simulink model "Brazoproject"  (R2013a)
settings: Solver=ode45  StartTime=0.0  StopTime=10.0  RelTol=1e-3
values from neighbouring files (symbols this model uses):
  m = [(m1*lc1^2)+m2*(l1^2+lc2^2+2*l1*lc2*cos(q2))+I1+I2 (m2*(lc2^2+l1*lc2*m2*cos(q2)+I2)) ... (first row only)    [brazomire.m]    (also in examvib3.m = 0.2533; fft estatica.m = [0:0.02:100]; fftestatica.m = [0:0.02:100])
undefined symbols (not defined in the file or in its folder): aumento, bacedymami, bacedymamixel, brazo1fribracarbono, brazo2frubra, Ensamblaje1, motordymamixel, par, Pieza1bASE, RootGround, RootPart, soporte, soporteM
libraries: mblibv1 x48
settings Model: Creator=Daniel  LastModifiedBy=Daniel
settings SimMechanicsCC: VisOnUpdateDiagram=on  VisDuringSimulation=on

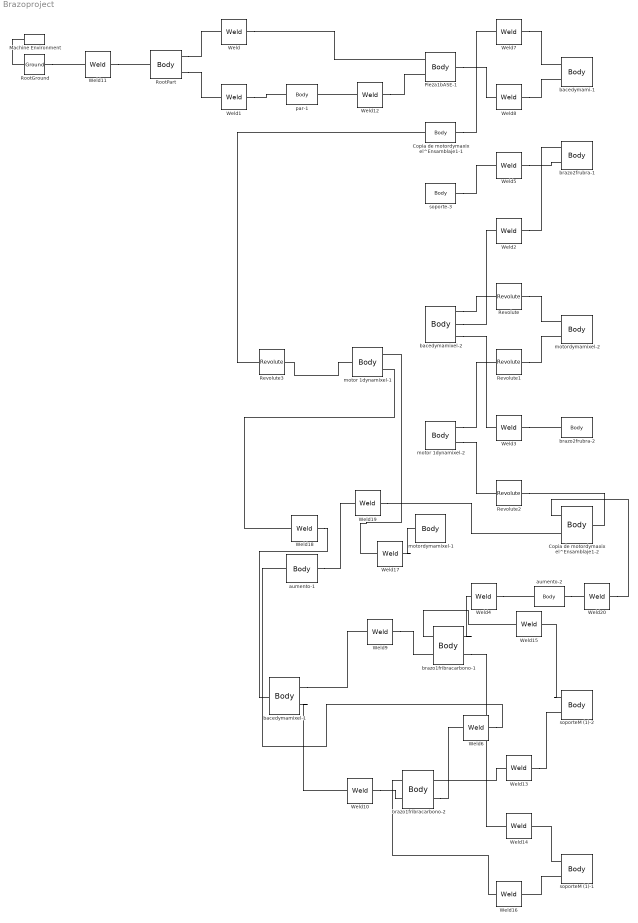
== system Brazoproject ==
  Copia de motordymaxixel^Ensamblaje1-1 : mblibv1/Bodies/Body  LConnTagsString=CS2  RConnTagsString=CS3  UpdateFromCAD=on  PMImportedID=Copia de motordymaxixel^Ensamblaje1-1  DialogClass=MechanicalBodyBlock  Mass=0.038592  MassUnits=kg  InertiaUnits=kg*m^2  Inertia=[1.11428e-05,-9.15437e-14,2.18753e-13;-9.15437e-14,6.03089e-06,1.38272e-07;2.18753e-13,1.38272e-07,9.55884e-06]  Shape=Cylinder  ShapeDims=[1 1]  ShapeUnits=m  ShapeUse=false  Density=1  DensityUnits=kg/m^3  DensityUse=false  GraphicsMode=GFXFILE  GraphicsFileName=Ensamblaje1 - Copia de motordymaxixel^Ensamblaje1-1.STL  BodyColorSelMode=COLORPALETTE  BodyColor=[1;0;0]  AttachedToCS=CS1  CG=Right$CG$[0.0211399 0.214749 0.233224]$WORLD$WORLD$m$[0 0 1;1 0 0;0 1 0]$3x3 Transform$rad$WORLD$false$Copia de motordymaxixel^Ensamblaje1-1::CG(AUTOGEN)  WorkingFrames=Right$CS1$[0.00471859 0.198749 0.20797]$WORLD$WORLD$m$[0 0 1;1 0 0;0 1 0]$3x3 Transform$rad$WORLD$false$Copia de motordymaxixel^Ensamblaje1-1::CS1(AUTOGEN)#Left$CS2$[0.0367186 0.214749 0.24647]$WORLD$WORLD$m$[1 0 0;0 1 0;0 0 1]$3x3 Transform$rad$WORLD$true$Copia de motordymaxixel^Ensamblaje1-1:-:motor 1dynamixel-1::Copia de motordymaxixel^Ensamblaje1-1(AUTOGEN)#Right$CS3$[0.00471859 0.222749 0.21047]$WORLD$WORLD$m$[1 0 0;0 1 0;0 0 1]$3x3 Transform$rad$WORLD$true$Copia de motordymaxixel^Ensamblaje1-1:-:bacedymami-1::Copia de motordymaxixel^Ensamblaje1-1(AUTOGEN)  CGPos=[0.0211399 0.214749 0.233224]  CGRot=[0 0 1;1 0 0;0 1 0]  CS0Pos=[]  CS0Rot=[]  CS1Pos=[0.00471859 0.198749 0.20797]  CS1Rot=[0 0 1;1 0 0;0 1 0]  CS2Pos=[0.0367186 0.214749 0.24647]  CS2Rot=[1 0 0;0 1 0;0 0 1]  CS3Pos=[0.00471859 0.222749 0.21047]  CS3Rot=[1 0 0;0 1 0;0 0 1]  CS4Pos=[]  CS4Rot=[]  CS5Pos=[]  CS5Rot=[]  CS6Pos=[]  CS6Rot=[]  CS7Pos=[]  CS7Rot=[]  CS8Pos=[]  CS8Rot=[]  CS9Pos=[]  CS9Rot=[]  CS10Pos=[]  CS10Rot=[]  CS11Pos=[]  CS11Rot=[]  CS12Pos=[]  CS12Rot=[]  CS13Pos=[]  CS13Rot=[]  CS14Pos=[]  CS14Rot=[]  CS15Pos=[]  CS15Rot=[]  CS16Pos=[]  CS16Rot=[]  CS17Pos=[]  CS17Rot=[]  CS18Pos=[]  CS18Rot=[]  CS19Pos=[]  CS19Rot=[]  CS20Pos=[]  CS20Rot=[]
  Copia de motordymaxixel^Ensamblaje1-2 : mblibv1/Bodies/Body  LConnTagsString=CS1|CS3  RConnTagsString=CS2  UpdateFromCAD=on  PMImportedID=Copia de motordymaxixel^Ensamblaje1-2  DialogClass=MechanicalBodyBlock  Mass=0.038592  MassUnits=kg  InertiaUnits=kg*m^2  Inertia=[1.11428e-05,-9.15437e-14,2.18753e-13;-9.15437e-14,6.03089e-06,1.38272e-07;2.18753e-13,1.38272e-07,9.55884e-06]  Shape=Cylinder  ShapeDims=[1 1]  ShapeUnits=m  ShapeUse=false  Density=1  DensityUnits=kg/m^3  DensityUse=false  GraphicsMode=GFXFILE  GraphicsFileName=Ensamblaje1 - Copia de motordymaxixel^Ensamblaje1-2.STL  BodyColorSelMode=COLORPALETTE  BodyColor=[1 0 0]  AttachedToCS=CS1  CG=Left$CG$[0.0201399 0.341824 0.297002]$WORLD$WORLD$m$[0 0 1;0.36951 0.929227 0;-0.929227 0.36951 0]$3x3 Transform$rad$WORLD$false$Copia de motordymaxixel^Ensamblaje1-2::CG(AUTOGEN)  WorkingFrames=Left$CS1$[0.00371859 0.312445 0.302538]$WORLD$WORLD$m$[0 0 1;0.36951 0.929227 0;-0.929227 0.36951 0]$3x3 Transform$rad$WORLD$true$Copia de motordymaxixel^Ensamblaje1-2::CS1(AUTOGEN)#Right$CS2$[0.0357186 0.354133 0.301897]$WORLD$WORLD$m$[1 0 0;0 1 0;0 0 1]$3x3 Transform$rad$WORLD$true$Copia de motordymaxixel^Ensamblaje1-2:-:motor 1dynamixel-2::Copia de motordymaxixel^Ensamblaje1-2(AUTOGEN)#Left$CS3$[0.00371859 0.198979 0.253651]$WORLD$WORLD$m$[1 0 0;0 1 0;0 0 1]$3x3 Transform$rad$WORLD$true$Copia de motordymaxixel^Ensamblaje1-2:-:aumento-1::Copia de motordymaxixel^Ensamblaje1-2(AUTOGEN)#Left$CS4$[0.00371859 0.317724 0.296028]$WORLD$WORLD$m$[1 0 0;0 1 0;0 0 1]$3x3 Transform$rad$WORLD$false$Copia de motordymaxixel^Ensamblaje1-2:-:brazo1fribracarbono-2::Copia de motordymaxixel^Ensamblaje1-2(AUTOGEN)  CGPos=[0.0201399 0.341824 0.297002]  CGRot=[0 0 1;0.36951 0.929227 0;-0.929227 0.36951 0]  CS0Pos=[]  CS0Rot=[]  CS1Pos=[0.00371859 0.312445 0.302538]  CS1Rot=[0 0 1;0.36951 0.929227 0;-0.929227 0.36951 0]  CS2Pos=[0.0357186 0.354133 0.301897]  CS2Rot=[1 0 0;0 1 0;0 0 1]  CS3Pos=[0.00371859 0.198979 0.253651]  CS3Rot=[1 0 0;0 1 0;0 0 1]  CS4Pos=[0.00371859 0.317724 0.296028]  CS4Rot=[1 0 0;0 1 0;0 0 1]  CS5Pos=[]  CS5Rot=[]  CS6Pos=[]  CS6Rot=[]  CS7Pos=[]  CS7Rot=[]  CS8Pos=[]  CS8Rot=[]  CS9Pos=[]  CS9Rot=[]  CS10Pos=[]  CS10Rot=[]  CS11Pos=[]  CS11Rot=[]  CS12Pos=[]  CS12Rot=[]  CS13Pos=[]  CS13Rot=[]  CS14Pos=[]  CS14Rot=[]  CS15Pos=[]  CS15Rot=[]  CS16Pos=[]  CS16Rot=[]  CS17Pos=[]  CS17Rot=[]  CS18Pos=[]  CS18Rot=[]  CS19Pos=[]  CS19Rot=[]  CS20Pos=[]  CS20Rot=[]
  Machine Environment : mblibv1/Bodies/Machine Environment  PortType=env  PhysicalDomain=Mechanical  DialogTemplateClass=MECH.MachineEnvironment  SyncWhenCopied=off  Gravity=[0 -9.81 0]  GravityUnits=m/s^2  GravityAsSignal=off  Dimensionality=Auto-detect  AnalysisType=Forward dynamics  LinearAssemblyTolerance=1e-3  LinearAssemblyToleranceUnits=m  AngularAssemblyTolerance=1e-3  AngularAssemblyToleranceUnits=rad  ConstraintSolverType=Machine precision  ConstraintRelTolerance=1e-4  ConstraintAbsTolerance=1e-4  UseRobustSingularityHandling=off  RedundancyAnalysisToleranceType=Automatically select tolerance  RedundancyAnalysisTolerance=1e-14  StatePerturbationType=Fixed  PerturbationSize=1e-5  VisualizeMachine=on  BodyVisualizationType=Use model default body geometries  BodyColorSelMode=Use model default  DefaultBodyColor=[1 0 0]
  Pieza1bASE-1 : mblibv1/Bodies/Body  LConnTagsString=CS2|CS4  RConnTagsString=CS3  UpdateFromCAD=on  PMImportedID=Pieza1bASE-1  DialogClass=MechanicalBodyBlock  Mass=0.00556696  MassUnits=kg  InertiaUnits=kg*m^2  Inertia=[4.51477e-07,0,0;0,5.93671e-06,0;0,0,6.38731e-06]  Shape=Cylinder  ShapeDims=[1 1]  ShapeUnits=m  ShapeUse=false  Density=1  DensityUnits=kg/m^3  DensityUse=false  GraphicsMode=GFXFILE  GraphicsFileName=Ensamblaje1 - Pieza1bASE-1.STL  BodyColorSelMode=COLORPALETTE  BodyColor=[0.74902 0 0.74902]  AttachedToCS=CS1  CG=Right$CG$[0.0207186 0.212333 0.203985]$WORLD$WORLD$m$[1 0 0;0 1 0;0 0 1]$3x3 Transform$rad$WORLD$false$Pieza1bASE-1::CG(AUTOGEN)  WorkingFrames=Right$CS1$[-0.0392814 0.212749 0.2035]$WORLD$WORLD$m$[1 0 0;0 1 0;0 0 1]$3x3 Transform$rad$WORLD$false$Pieza1bASE-1::CS1(AUTOGEN)#Left$CS2$[0.0207186 0.212333 0.203985]$WORLD$WORLD$m$[1 0 0;0 1 0;0 0 1]$3x3 Transform$rad$WORLD$true$Ensamblaje1/RootPart:-:Pieza1bASE-1::Pieza1bASE-1(AUTOGEN)#Right$CS3$[0.0127186 0.223249 0.20447]$WORLD$WORLD$m$[1 0 0;0 1 0;0 0 1]$3x3 Transform$rad$WORLD$true$Pieza1bASE-1:-:bacedymami-1::Pieza1bASE-1(AUTOGEN)#Left$CS4$[-0.0342814 0.200749 0.2035]$WORLD$WORLD$m$[1 0 0;0 1 0;0 0 1]$3x3 Transform$rad$WORLD$true$Pieza1bASE-1:-:par-1::Pieza1bASE-1(AUTOGEN)  CGPos=[0.0207186 0.212333 0.203985]  CGRot=[1 0 0;0 1 0;0 0 1]  CS0Pos=[]  CS0Rot=[]  CS1Pos=[-0.0392814 0.212749 0.2035]  CS1Rot=[1 0 0;0 1 0;0 0 1]  CS2Pos=[0.0207186 0.212333 0.203985]  CS2Rot=[1 0 0;0 1 0;0 0 1]  CS3Pos=[0.0127186 0.223249 0.20447]  CS3Rot=[1 0 0;0 1 0;0 0 1]  CS4Pos=[-0.0342814 0.200749 0.2035]  CS4Rot=[1 0 0;0 1 0;0 0 1]  CS5Pos=[]  CS5Rot=[]  CS6Pos=[]  CS6Rot=[]  CS7Pos=[]  CS7Rot=[]  CS8Pos=[]  CS8Rot=[]  CS9Pos=[]  CS9Rot=[]  CS10Pos=[]  CS10Rot=[]  CS11Pos=[]  CS11Rot=[]  CS12Pos=[]  CS12Rot=[]  CS13Pos=[]  CS13Rot=[]  CS14Pos=[]  CS14Rot=[]  CS15Pos=[]  CS15Rot=[]  CS16Pos=[]  CS16Rot=[]  CS17Pos=[]  CS17Rot=[]  CS18Pos=[]  CS18Rot=[]  CS19Pos=[]  CS19Rot=[]  CS20Pos=[]  CS20Rot=[]
  Revolute : mblibv1/Joints/Revolute  LConnTagsString=__newl0  RConnTagsString=__newr0  UpdateFromCAD=on  PMImportedID=bacedymamixel-2:-:motordymamixel-2  NumSAPorts=0  CutJoint=off  MarkAsCut=off  Primitives=prismatic  PrimitiveProps=R1$WORLD$[1,0,0]$revolute  DialogClass=JointBlock  R1Axis=[1,0,0]
  Revolute1 : mblibv1/Joints/Revolute  LConnTagsString=__newl0  RConnTagsString=__newr0  UpdateFromCAD=on  PMImportedID=motor 1dynamixel-2:-:motordymamixel-2  NumSAPorts=0  CutJoint=off  MarkAsCut=off  Primitives=prismatic  PrimitiveProps=R1$WORLD$[1,0,0]$revolute  DialogClass=JointBlock  R1Axis=[1,0,0]
  Revolute2 : mblibv1/Joints/Revolute  LConnTagsString=__newl0  RConnTagsString=__newr0  UpdateFromCAD=on  PMImportedID=Copia de motordymaxixel^Ensamblaje1-2:-:motor 1dynamixel-2  NumSAPorts=0  CutJoint=off  MarkAsCut=off  Primitives=prismatic  PrimitiveProps=R1$WORLD$[1,0,0]$revolute  DialogClass=JointBlock  R1Axis=[1,0,0]
  Revolute3 : mblibv1/Joints/Revolute  LConnTagsString=__newl0  RConnTagsString=__newr0  UpdateFromCAD=on  PMImportedID=Copia de motordymaxixel^Ensamblaje1-1:-:motor 1dynamixel-1  NumSAPorts=0  CutJoint=off  MarkAsCut=off  Primitives=prismatic  PrimitiveProps=R1$World$[1,0,0]$revolute  DialogClass=JointBlock  R1Axis=[1,0,0]
  RootGround : mblibv1/Bodies/Ground  UpdateFromCAD=on  PMImportedID=RootGround  LeftPortType=env  RightPortType=workingframe  PhysicalDomain=Mechanical  DialogClass=GroundBlock  CoordPosition=[0.0202975,0.248993,0.241749]  CoordPositionUnits=m  StateVectorMgrId=1  MachineId=[0 0]  ShowEnvPort=on
  RootPart : mblibv1/Bodies/Body  LConnTagsString=CS4  RConnTagsString=CS2|CS3  UpdateFromCAD=on  PMImportedID=Ensamblaje1/RootPart  DialogClass=MechanicalBodyBlock  Mass=0  MassUnits=kg  InertiaUnits=kg*m^2  Inertia=[0,0,0;0,0,0;0,0,0]  Shape=Cylinder  ShapeDims=[1 1]  ShapeUnits=m  ShapeUse=false  Density=1  DensityUnits=kg/m^3  DensityUse=false  GraphicsMode=MACHINE_DEFAULT  BodyColorSelMode=MACHINE_DEFAULT  BodyColor=[1 0 0]  AttachedToCS=CS1  CG=Right$CG$[0.0202975 0.248993 0.241749]$WORLD$WORLD$m$[1 0 0;0 1 0;0 0 1]$3x3 Transform$rad$WORLD$false$Ensamblaje1/RootPart::CG(AUTOGEN)  WorkingFrames=Right$CS1$[0 0 0]$WORLD$WORLD$m$[1 0 0;0 1 0;0 0 1]$3x3 Transform$rad$WORLD$false$Ensamblaje1/RootPart::CS1(AUTOGEN)#Right$CS2$[0.0207186 0.212333 0.203985]$WORLD$WORLD$m$[1 0 0;0 1 0;0 0 1]$3x3 Transform$rad$WORLD$true$Ensamblaje1/RootPart:-:Pieza1bASE-1::Ensamblaje1/RootPart(AUTOGEN)#Right$CS3$[0.0217437 0.176811 0.202]$WORLD$WORLD$m$[1 0 0;0 1 0;0 0 1]$3x3 Transform$rad$WORLD$true$Ensamblaje1/RootPart:-:par-1::Ensamblaje1/RootPart(AUTOGEN)#Left$CS4$[0.0202975 0.248993 0.241749]$WORLD$WORLD$m$[1 0 0;0 1 0;0 0 1]$3x3 Transform$rad$WORLD$true$Ensamblaje1/RootPart:-:RootGround::Ensamblaje1/RootPart(AUTOGEN)  CGPos=[0.0202975 0.248993 0.241749]  CGRot=[1 0 0;0 1 0;0 0 1]  CS0Pos=[]  CS0Rot=[]  CS1Pos=[0 0 0]  CS1Rot=[1 0 0;0 1 0;0 0 1]  CS2Pos=[0.0207186 0.212333 0.203985]  CS2Rot=[1 0 0;0 1 0;0 0 1]  CS3Pos=[0.0217437 0.176811 0.202]  CS3Rot=[1 0 0;0 1 0;0 0 1]  CS4Pos=[0.0202975 0.248993 0.241749]  CS4Rot=[1 0 0;0 1 0;0 0 1]  CS5Pos=[]  CS5Rot=[]  CS6Pos=[]  CS6Rot=[]  CS7Pos=[]  CS7Rot=[]  CS8Pos=[]  CS8Rot=[]  CS9Pos=[]  CS9Rot=[]  CS10Pos=[]  CS10Rot=[]  CS11Pos=[]  CS11Rot=[]  CS12Pos=[]  CS12Rot=[]  CS13Pos=[]  CS13Rot=[]  CS14Pos=[]  CS14Rot=[]  CS15Pos=[]  CS15Rot=[]  CS16Pos=[]  CS16Rot=[]  CS17Pos=[]  CS17Rot=[]  CS18Pos=[]  CS18Rot=[]  CS19Pos=[]  CS19Rot=[]  CS20Pos=[]  CS20Rot=[]
  Weld : mblibv1/Joints/Weld  LConnTagsString=__newl0  RConnTagsString=__newr0  UpdateFromCAD=on  PMImportedID=Ensamblaje1/RootPart:-:Pieza1bASE-1  NumSAPorts=0  CutJoint=off  MarkAsCut=off  Primitives=weld  PrimitiveProps=W$WORLD$[0.57735,0.57735,0.57735]$weld  DialogClass=JointBlock  WAxis=[0.57735,0.57735,0.57735]
  Weld1 : mblibv1/Joints/Weld  LConnTagsString=__newl0  RConnTagsString=__newr0  UpdateFromCAD=on  PMImportedID=Ensamblaje1/RootPart:-:par-1  NumSAPorts=0  CutJoint=off  MarkAsCut=off  Primitives=weld  PrimitiveProps=W$WORLD$[0.57735,0.57735,0.57735]$weld  DialogClass=JointBlock  WAxis=[0.57735,0.57735,0.57735]
  Weld10 : mblibv1/Joints/Weld  LConnTagsString=__newl0  RConnTagsString=__newr0  UpdateFromCAD=on  PMImportedID=bacedymamixel-1:-:brazo1fribracarbono-2  NumSAPorts=0  CutJoint=off  MarkAsCut=off  Primitives=weld  PrimitiveProps=W$WORLD$[0.57735,0.57735,0.57735]$weld  DialogClass=JointBlock  WAxis=[0.57735,0.57735,0.57735]
  Weld11 : mblibv1/Joints/Weld  LConnTagsString=__newl0  RConnTagsString=__newr0  UpdateFromCAD=on  PMImportedID=Ensamblaje1/RootPart:-:RootGround  NumSAPorts=0  CutJoint=off  MarkAsCut=off  Primitives=weld  PrimitiveProps=W$WORLD$[0.57735,0.57735,0.57735]$weld  DialogClass=JointBlock  WAxis=[0.57735,0.57735,0.57735]
  Weld12 : mblibv1/Joints/Weld  LConnTagsString=__newl0  RConnTagsString=__newr0  UpdateFromCAD=on  NumSAPorts=0  CutJoint=off  MarkAsCut=off  Primitives=weld  PrimitiveProps=W$World$[0.57735,0.57735,0.57735]$weld  DialogClass=JointBlock  WAxis=[0.57735,0.57735,0.57735]
  Weld{4,13..20} (9 alike) : mblibv1/Joints/Weld  LConnTagsString=__newl0  RConnTagsString=__newr0  UpdateFromCAD=on  NumSAPorts=0  CutJoint=off  MarkAsCut=off  Primitives=weld  PrimitiveProps=W$WORLD$[0.57735,0.57735,0.57735]$weld  DialogClass=JointBlock  WAxis=[0.57735,0.57735,0.57735]
  Weld2 : mblibv1/Joints/Weld  LConnTagsString=__newl0  RConnTagsString=__newr0  UpdateFromCAD=on  PMImportedID=bacedymamixel-2:-:brazo2frubra-1  NumSAPorts=0  CutJoint=off  MarkAsCut=off  Primitives=weld  PrimitiveProps=W$WORLD$[0.57735,0.57735,0.57735]$weld  DialogClass=JointBlock  WAxis=[0.57735,0.57735,0.57735]
  Weld3 : mblibv1/Joints/Weld  LConnTagsString=__newl0  RConnTagsString=__newr0  UpdateFromCAD=on  PMImportedID=bacedymamixel-2:-:brazo2frubra-2  NumSAPorts=0  CutJoint=off  MarkAsCut=off  Primitives=weld  PrimitiveProps=W$WORLD$[0.57735,0.57735,0.57735]$weld  DialogClass=JointBlock  WAxis=[0.57735,0.57735,0.57735]
  Weld5 : mblibv1/Joints/Weld  LConnTagsString=__newl0  RConnTagsString=__newr0  UpdateFromCAD=on  PMImportedID=brazo2frubra-1:-:soporte-3  NumSAPorts=0  CutJoint=off  MarkAsCut=off  Primitives=weld  PrimitiveProps=W$WORLD$[0.57735,0.57735,0.57735]$weld  DialogClass=JointBlock  WAxis=[0.57735,0.57735,0.57735]
  Weld6 : mblibv1/Joints/Weld  LConnTagsString=__newl0  RConnTagsString=__newr0  UpdateFromCAD=on  PMImportedID=aumento-1:-:brazo1fribracarbono-2  NumSAPorts=0  CutJoint=off  MarkAsCut=off  Primitives=weld  PrimitiveProps=W$WORLD$[0.57735,0.57735,0.57735]$weld  DialogClass=JointBlock  WAxis=[0.57735,0.57735,0.57735]
  Weld7 : mblibv1/Joints/Weld  LConnTagsString=__newl0  RConnTagsString=__newr0  UpdateFromCAD=on  PMImportedID=Copia de motordymaxixel^Ensamblaje1-1:-:bacedymami-1  NumSAPorts=0  CutJoint=off  MarkAsCut=off  Primitives=weld  PrimitiveProps=W$World$[0.57735,0.57735,0.57735]$weld  DialogClass=JointBlock  WAxis=[0.57735,0.57735,0.57735]
  Weld8 : mblibv1/Joints/Weld  LConnTagsString=__newl0  RConnTagsString=__newr0  UpdateFromCAD=on  PMImportedID=Pieza1bASE-1:-:bacedymami-1  NumSAPorts=0  CutJoint=off  MarkAsCut=off  Primitives=weld  PrimitiveProps=W$World$[0.57735,0.57735,0.57735]$weld  DialogClass=JointBlock  WAxis=[0.57735,0.57735,0.57735]
  Weld9 : mblibv1/Joints/Weld  LConnTagsString=__newl0  RConnTagsString=__newr0  UpdateFromCAD=on  PMImportedID=bacedymamixel-1:-:brazo1fribracarbono-1  NumSAPorts=0  CutJoint=off  MarkAsCut=off  Primitives=weld  PrimitiveProps=W$WORLD$[0.57735,0.57735,0.57735]$weld  DialogClass=JointBlock  WAxis=[0.57735,0.57735,0.57735]
  aumento-1 : mblibv1/Bodies/Body  LConnTagsString=CS3  RConnTagsString=CS2  UpdateFromCAD=on  PMImportedID=aumento-1  DialogClass=MechanicalBodyBlock  Mass=0.0041092  MassUnits=kg  InertiaUnits=kg*m^2  Inertia=[5.38714e-07,0,0;0,6.96458e-07,0;0,0,2.01575e-07]  Shape=Cylinder  ShapeDims=[1 1]  ShapeUnits=m  ShapeUse=false  Density=1  DensityUnits=kg/m^3  DensityUse=false  GraphicsMode=GFXFILE  GraphicsFileName=Ensamblaje1 - aumento-1.STL  BodyColorSelMode=COLORPALETTE  BodyColor=[0 1 0]  AttachedToCS=CS1  CG=Right$CG$[-0.00028141 0.322902 0.289478]$WORLD$WORLD$m$[0 -1 0;0.929227 0 -0.36951;0.36951 0 0.929227]$3x3 Transform$rad$WORLD$false$aumento-1::CG(AUTOGEN)  WorkingFrames=Right$CS1$[0.00371859 0.198979 0.253651]$WORLD$WORLD$m$[0 -1 0;0.929227 0 -0.36951;0.36951 0 0.929227]$3x3 Transform$rad$WORLD$false$aumento-1::CS1(AUTOGEN)#Right$CS2$[0.00371859 0.198979 0.253651]$WORLD$WORLD$m$[1 0 0;0 1 0;0 0 1]$3x3 Transform$rad$WORLD$true$Copia de motordymaxixel^Ensamblaje1-2:-:aumento-1::aumento-1(AUTOGEN)#Left$CS3$[-0.00428141 0.198979 0.253651]$WORLD$WORLD$m$[1 0 0;0 1 0;0 0 1]$3x3 Transform$rad$WORLD$true$aumento-1:-:brazo1fribracarbono-2::aumento-1(AUTOGEN)  CGPos=[-0.00028141 0.322902 0.289478]  CGRot=[0 -1 0;0.929227 0 -0.36951;0.36951 0 0.929227]  CS0Pos=[]  CS0Rot=[]  CS1Pos=[0.00371859 0.198979 0.253651]  CS1Rot=[0 -1 0;0.929227 0 -0.36951;0.36951 0 0.929227]  CS2Pos=[0.00371859 0.198979 0.253651]  CS2Rot=[1 0 0;0 1 0;0 0 1]  CS3Pos=[-0.00428141 0.198979 0.253651]  CS3Rot=[1 0 0;0 1 0;0 0 1]  CS4Pos=[]  CS4Rot=[]  CS5Pos=[]  CS5Rot=[]  CS6Pos=[]  CS6Rot=[]  CS7Pos=[]  CS7Rot=[]  CS8Pos=[]  CS8Rot=[]  CS9Pos=[]  CS9Rot=[]  CS10Pos=[]  CS10Rot=[]  CS11Pos=[]  CS11Rot=[]  CS12Pos=[]  CS12Rot=[]  CS13Pos=[]  CS13Rot=[]  CS14Pos=[]  CS14Rot=[]  CS15Pos=[]  CS15Rot=[]  CS16Pos=[]  CS16Rot=[]  CS17Pos=[]  CS17Rot=[]  CS18Pos=[]  CS18Rot=[]  CS19Pos=[]  CS19Rot=[]  CS20Pos=[]  CS20Rot=[]
  aumento-2 : mblibv1/Bodies/Body  LConnTagsString=CS2  RConnTagsString=CS1  UpdateFromCAD=on  PMImportedID=aumento-2  DialogClass=MechanicalBodyBlock  Mass=0.0041092  MassUnits=kg  InertiaUnits=kg*m^2  Inertia=[5.38714e-07,0,0;0,6.96458e-07,0;0,0,2.01575e-07]  Shape=Cylinder  ShapeDims=[1 1]  ShapeUnits=m  ShapeUse=false  Density=1  DensityUnits=kg/m^3  DensityUse=false  GraphicsMode=GFXFILE  GraphicsFileName=Ensamblaje1 - aumento-2.STL  BodyColorSelMode=COLORPALETTE  BodyColor=[0 1 0]  AttachedToCS=CS1  CG=Right$CG$[0.0397186 0.322902 0.289478]$WORLD$WORLD$m$[0 -1 0;0.929227 0 -0.36951;0.36951 0 0.929227]$3x3 Transform$rad$WORLD$false$aumento-2::CG(AUTOGEN)  WorkingFrames=Right$CS1$[0.0437186 0.198979 0.253651]$WORLD$WORLD$m$[0 -1 0;0.929227 0 -0.36951;0.36951 0 0.929227]$3x3 Transform$rad$WORLD$true$aumento-2::CS1(AUTOGEN)#Left$CS2$[0.0437186 0.208217 0.230421]$WORLD$WORLD$m$[1 0 0;0 1 0;0 0 1]$3x3 Transform$rad$WORLD$true$aumento-2:-:brazo1fribracarbono-1::aumento-2(AUTOGEN)  CGPos=[0.0397186 0.322902 0.289478]  CGRot=[0 -1 0;0.929227 0 -0.36951;0.36951 0 0.929227]  CS0Pos=[]  CS0Rot=[]  CS1Pos=[0.0437186 0.198979 0.253651]  CS1Rot=[0 -1 0;0.929227 0 -0.36951;0.36951 0 0.929227]  CS2Pos=[0.0437186 0.208217 0.230421]  CS2Rot=[1 0 0;0 1 0;0 0 1]  CS3Pos=[]  CS3Rot=[]  CS4Pos=[]  CS4Rot=[]  CS5Pos=[]  CS5Rot=[]  CS6Pos=[]  CS6Rot=[]  CS7Pos=[]  CS7Rot=[]  CS8Pos=[]  CS8Rot=[]  CS9Pos=[]  CS9Rot=[]  CS10Pos=[]  CS10Rot=[]  CS11Pos=[]  CS11Rot=[]  CS12Pos=[]  CS12Rot=[]  CS13Pos=[]  CS13Rot=[]  CS14Pos=[]  CS14Rot=[]  CS15Pos=[]  CS15Rot=[]  CS16Pos=[]  CS16Rot=[]  CS17Pos=[]  CS17Rot=[]  CS18Pos=[]  CS18Rot=[]  CS19Pos=[]  CS19Rot=[]  CS20Pos=[]  CS20Rot=[]
  bacedymami-1 : mblibv1/Bodies/Body  LConnTagsString=CS2|CS3  UpdateFromCAD=on  PMImportedID=bacedymami-1  DialogClass=MechanicalBodyBlock  Mass=0.00364977  MassUnits=kg  InertiaUnits=kg*m^2  Inertia=[2.2798e-07,0,0;0,7.22927e-07,0;0,0,5.18505e-07]  Shape=Cylinder  ShapeDims=[1 1]  ShapeUnits=m  ShapeUse=false  Density=1  DensityUnits=kg/m^3  DensityUse=false  GraphicsMode=GFXFILE  GraphicsFileName=Ensamblaje1 - bacedymami-1.STL  BodyColorSelMode=COLORPALETTE  BodyColor=[0 0 1]  AttachedToCS=CS1  CG=Right$CG$[0.0207186 0.214749 0.206996]$WORLD$WORLD$m$[1 0 0;0 0 1;0 -1 0]$3x3 Transform$rad$WORLD$false$bacedymami-1::CG(AUTOGEN)  WorkingFrames=Right$CS1$[0.00171859 0.202249 0.21347]$WORLD$WORLD$m$[1 0 0;0 0 1;0 -1 0]$3x3 Transform$rad$WORLD$false$bacedymami-1::CS1(AUTOGEN)#Left$CS2$[0.00471859 0.222749 0.21047]$WORLD$WORLD$m$[1 0 0;0 1 0;0 0 1]$3x3 Transform$rad$WORLD$true$Copia de motordymaxixel^Ensamblaje1-1:-:bacedymami-1::bacedymami-1(AUTOGEN)#Left$CS3$[0.0127186 0.223249 0.20447]$WORLD$WORLD$m$[1 0 0;0 1 0;0 0 1]$3x3 Transform$rad$WORLD$true$Pieza1bASE-1:-:bacedymami-1::bacedymami-1(AUTOGEN)  CGPos=[0.0207186 0.214749 0.206996]  CGRot=[1 0 0;0 0 1;0 -1 0]  CS0Pos=[]  CS0Rot=[]  CS1Pos=[0.00171859 0.202249 0.21347]  CS1Rot=[1 0 0;0 0 1;0 -1 0]  CS2Pos=[0.00471859 0.222749 0.21047]  CS2Rot=[1 0 0;0 1 0;0 0 1]  CS3Pos=[0.0127186 0.223249 0.20447]  CS3Rot=[1 0 0;0 1 0;0 0 1]  CS4Pos=[]  CS4Rot=[]  CS5Pos=[]  CS5Rot=[]  CS6Pos=[]  CS6Rot=[]  CS7Pos=[]  CS7Rot=[]  CS8Pos=[]  CS8Rot=[]  CS9Pos=[]  CS9Rot=[]  CS10Pos=[]  CS10Rot=[]  CS11Pos=[]  CS11Rot=[]  CS12Pos=[]  CS12Rot=[]  CS13Pos=[]  CS13Rot=[]  CS14Pos=[]  CS14Rot=[]  CS15Pos=[]  CS15Rot=[]  CS16Pos=[]  CS16Rot=[]  CS17Pos=[]  CS17Rot=[]  CS18Pos=[]  CS18Rot=[]  CS19Pos=[]  CS19Rot=[]  CS20Pos=[]  CS20Rot=[]
  bacedymamixel-1 : mblibv1/Bodies/Body  LConnTagsString=CS3  RConnTagsString=CS2|CS4  UpdateFromCAD=on  PMImportedID=bacedymamixel-1  DialogClass=MechanicalBodyBlock  Mass=0.0121791  MassUnits=kg  InertiaUnits=kg*m^2  Inertia=[1.98007e-06,0,-1.40111e-10;0,4.46715e-06,6.99395e-11;-1.40111e-10,6.99395e-11,5.19045e-06]  Shape=Cylinder  ShapeDims=[1 1]  ShapeUnits=m  ShapeUse=false  Density=1  DensityUnits=kg/m^3  DensityUse=false  GraphicsMode=GFXFILE  GraphicsFileName=Ensamblaje1 - bacedymamixel-1.STL  BodyColorSelMode=COLORPALETTE  BodyColor=[0 0 1]  AttachedToCS=CS1  CG=Right$CG$[0.0197186 0.22777 0.251647]$WORLD$WORLD$m$[1 0 0;0 0.929227 -0.36951;0 0.36951 0.929227]$3x3 Transform$rad$WORLD$false$bacedymamixel-1::CG(AUTOGEN)  WorkingFrames=Right$CS1$[-0.00428141 0.208217 0.230421]$WORLD$WORLD$m$[1 0 0;0 0.929227 -0.36951;0 0.36951 0.929227]$3x3 Transform$rad$WORLD$false$bacedymamixel-1::CS1(AUTOGEN)#Right$CS2$[0.0437186 0.233361 0.267323]$WORLD$WORLD$m$[1 0 0;0 1 0;0 0 1]$3x3 Transform$rad$WORLD$true$bacedymamixel-1:-:brazo1fribracarbono-1::bacedymamixel-1(AUTOGEN)#Left$CS3$[-0.00028141 0.214749 0.24647]$WORLD$WORLD$m$[1 0 0;0 1 0;0 0 1]$3x3 Transform$rad$WORLD$true$bacedymamixel-1:-:motordymamixel-1::bacedymamixel-1(AUTOGEN)#Right$CS4$[-0.00428141 0.198979 0.253651]$WORLD$WORLD$m$[1 0 0;0 1 0;0 0 1]$3x3 Transform$rad$WORLD$true$bacedymamixel-1:-:brazo1fribracarbono-2::bacedymamixel-1(AUTOGEN)  CGPos=[0.0197186 0.22777 0.251647]  CGRot=[1 0 0;0 0.929227 -0.36951;0 0.36951 0.929227]  CS0Pos=[]  CS0Rot=[]  CS1Pos=[-0.00428141 0.208217 0.230421]  CS1Rot=[1 0 0;0 0.929227 -0.36951;0 0.36951 0.929227]  CS2Pos=[0.0437186 0.233361 0.267323]  CS2Rot=[1 0 0;0 1 0;0 0 1]  CS3Pos=[-0.00028141 0.214749 0.24647]  CS3Rot=[1 0 0;0 1 0;0 0 1]  CS4Pos=[-0.00428141 0.198979 0.253651]  CS4Rot=[1 0 0;0 1 0;0 0 1]  CS5Pos=[]  CS5Rot=[]  CS6Pos=[]  CS6Rot=[]  CS7Pos=[]  CS7Rot=[]  CS8Pos=[]  CS8Rot=[]  CS9Pos=[]  CS9Rot=[]  CS10Pos=[]  CS10Rot=[]  CS11Pos=[]  CS11Rot=[]  CS12Pos=[]  CS12Rot=[]  CS13Pos=[]  CS13Rot=[]  CS14Pos=[]  CS14Rot=[]  CS15Pos=[]  CS15Rot=[]  CS16Pos=[]  CS16Rot=[]  CS17Pos=[]  CS17Rot=[]  CS18Pos=[]  CS18Rot=[]  CS19Pos=[]  CS19Rot=[]  CS20Pos=[]  CS20Rot=[]
  bacedymamixel-2 : mblibv1/Bodies/Body  RConnTagsString=CS2|CS3|CS4  UpdateFromCAD=on  PMImportedID=bacedymamixel-2  DialogClass=MechanicalBodyBlock  Mass=0.0121791  MassUnits=kg  InertiaUnits=kg*m^2  Inertia=[1.98007e-06,0,-1.40111e-10;0,4.46715e-06,6.99395e-11;-1.40111e-10,6.99395e-11,5.19045e-06]  Shape=Cylinder  ShapeDims=[1 1]  ShapeUnits=m  ShapeUse=false  Density=1  DensityUnits=kg/m^3  DensityUse=false  GraphicsMode=GFXFILE  GraphicsFileName=Ensamblaje1 - bacedymamixel-2.STL  BodyColorSelMode=COLORPALETTE  BodyColor=[0 0 1]  AttachedToCS=CS1  CG=Right$CG$[0.0187186 0.361419 0.289927]$WORLD$WORLD$m$[1 0 0;0 0.520016 0.854156;0 -0.854156 0.520016]$3x3 Transform$rad$WORLD$false$bacedymamixel-2::CG(AUTOGEN)  WorkingFrames=Right$CS1$[-0.00528141 0.337216 0.305646]$WORLD$WORLD$m$[1 0 0;0 0.520016 0.854156;0 -0.854156 0.520016]$3x3 Transform$rad$WORLD$false$bacedymamixel-2::CS1(AUTOGEN)#Right$CS2$[-0.00128141 0.354133 0.301897]$WORLD$WORLD$m$[1 0 0;0 1 0;0 0 1]$3x3 Transform$rad$WORLD$true$bacedymamixel-2:-:motordymamixel-2::bacedymamixel-2(AUTOGEN)#Right$CS3$[-0.00528141 0.358569 0.318647]$WORLD$WORLD$m$[1 0 0;0 1 0;0 0 1]$3x3 Transform$rad$WORLD$true$bacedymamixel-2:-:brazo2frubra-1::bacedymamixel-2(AUTOGEN)#Right$CS4$[0.0427186 0.37781 0.287043]$WORLD$WORLD$m$[1 0 0;0 1 0;0 0 1]$3x3 Transform$rad$WORLD$true$bacedymamixel-2:-:brazo2frubra-2::bacedymamixel-2(AUTOGEN)  CGPos=[0.0187186 0.361419 0.289927]  CGRot=[1 0 0;0 0.520016 0.854156;0 -0.854156 0.520016]  CS0Pos=[]  CS0Rot=[]  CS1Pos=[-0.00528141 0.337216 0.305646]  CS1Rot=[1 0 0;0 0.520016 0.854156;0 -0.854156 0.520016]  CS2Pos=[-0.00128141 0.354133 0.301897]  CS2Rot=[1 0 0;0 1 0;0 0 1]  CS3Pos=[-0.00528141 0.358569 0.318647]  CS3Rot=[1 0 0;0 1 0;0 0 1]  CS4Pos=[0.0427186 0.37781 0.287043]  CS4Rot=[1 0 0;0 1 0;0 0 1]  CS5Pos=[]  CS5Rot=[]  CS6Pos=[]  CS6Rot=[]  CS7Pos=[]  CS7Rot=[]  CS8Pos=[]  CS8Rot=[]  CS9Pos=[]  CS9Rot=[]  CS10Pos=[]  CS10Rot=[]  CS11Pos=[]  CS11Rot=[]  CS12Pos=[]  CS12Rot=[]  CS13Pos=[]  CS13Rot=[]  CS14Pos=[]  CS14Rot=[]  CS15Pos=[]  CS15Rot=[]  CS16Pos=[]  CS16Rot=[]  CS17Pos=[]  CS17Rot=[]  CS18Pos=[]  CS18Rot=[]  CS19Pos=[]  CS19Rot=[]  CS20Pos=[]  CS20Rot=[]
  brazo1fribracarbono-1 : mblibv1/Bodies/Body  LConnTagsString=CS3|CS5  RConnTagsString=CS2|CS4  UpdateFromCAD=on  PMImportedID=brazo1fribracarbono-1  DialogClass=MechanicalBodyBlock  Mass=0.00772701  MassUnits=kg  InertiaUnits=kg*m^2  Inertia=[7.39171e-07,0,0;0,1.43285e-05,0;0,0,1.35906e-05]  Shape=Cylinder  ShapeDims=[1 1]  ShapeUnits=m  ShapeUse=false  Density=1  DensityUnits=kg/m^3  DensityUse=false  GraphicsMode=GFXFILE  GraphicsFileName=Ensamblaje1 - brazo1fribracarbono-1.STL  BodyColorSelMode=COLORPALETTE  BodyColor=[0 0.49804 0]  AttachedToCS=CS1  CG=Left$CG$[0.0442036 0.271763 0.269142]$Adjoining$Adjoining$m$[0 1 0;0.929227 0 0.36951;0.36951 0 -0.929227]$3x3 Transform$rad$WORLD$false$brazo1fribracarbono-1::CG(AUTOGEN)  WorkingFrames=Right$CS1$[0.0437186 0.208217 0.230421]$Adjoining$Adjoining$m$[0 1 0;0.929227 0 0.36951;0.36951 0 -0.929227]$3x3 Transform$rad$WORLD$false$brazo1fribracarbono-1::CS1(AUTOGEN)#Right$CS2$[0.0437186 0.208217 0.230421]$Adjoining$Adjoining$m$[1 0 0;0 1 0;0 0 1]$3x3 Transform$rad$Adjoining$true$aumento-2:-:brazo1fribracarbono-1::brazo1fribracarbono-1(AUTOGEN)#Left$CS3$[0.0437186 0.275085 0.261853]$Adjoining$Adjoining$m$[1 0 0;0 1 0;0 0 1]$3x3 Transform$rad$Adjoining$true$brazo1fribracarbono-1:-:soporteM (1)-2::brazo1fribracarbono-1(AUTOGEN)#Right$CS4$[0.0437186 0.208217 0.230421]$Adjoining$Adjoining$m$[1 0 0;0 1 0;0 0 1]$3x3 Transform$rad$Adjoining$true$brazo1fribracarbono-1:-:soporteM (1)-1::brazo1fribracarbono-1(AUTOGEN)#Left$CS5$[0.0437186 0.233361 0.267323]$Adjoining$Adjoining$m$[1 0 0;0 1 0;0 0 1]$3x3 Transform$rad$Adjoining$true$bacedymamixel-1:-:brazo1fribracarbono-1::brazo1fribracarbono-1(AUTOGEN)  CGPos=[0.0442036 0.271763 0.269142]  CGRot=[0 1 0;0.929227 0 0.36951;0.36951 0 -0.929227]  CS0Pos=[]  CS0Rot=[]  CS1Pos=[0.0437186 0.208217 0.230421]  CS1Rot=[0 1 0;0.929227 0 0.36951;0.36951 0 -0.929227]  CS2Pos=[0.0437186 0.208217 0.230421]  CS2Rot=[1 0 0;0 1 0;0 0 1]  CS3Pos=[0.0437186 0.275085 0.261853]  CS3Rot=[1 0 0;0 1 0;0 0 1]  CS4Pos=[0.0437186 0.208217 0.230421]  CS4Rot=[1 0 0;0 1 0;0 0 1]  CS5Pos=[0.0437186 0.233361 0.267323]  CS5Rot=[1 0 0;0 1 0;0 0 1]  CS6Pos=[]  CS6Rot=[]  CS7Pos=[]  CS7Rot=[]  CS8Pos=[]  CS8Rot=[]  CS9Pos=[]  CS9Rot=[]  CS10Pos=[]  CS10Rot=[]  CS11Pos=[]  CS11Rot=[]  CS12Pos=[]  CS12Rot=[]  CS13Pos=[]  CS13Rot=[]  CS14Pos=[]  CS14Rot=[]  CS15Pos=[]  CS15Rot=[]  CS16Pos=[]  CS16Rot=[]  CS17Pos=[]  CS17Rot=[]  CS18Pos=[]  CS18Rot=[]  CS19Pos=[]  CS19Rot=[]  CS20Pos=[]  CS20Rot=[]
  brazo1fribracarbono-2 : mblibv1/Bodies/Body  LConnTagsString=CS5|CS6  RConnTagsString=CS3|CS4  UpdateFromCAD=on  PMImportedID=brazo1fribracarbono-2  DialogClass=MechanicalBodyBlock  Mass=0.00772701  MassUnits=kg  InertiaUnits=kg*m^2  Inertia=[7.39171e-07,0,0;0,1.43285e-05,0;0,0,1.35906e-05]  Shape=Cylinder  ShapeDims=[1 1]  ShapeUnits=m  ShapeUse=false  Density=1  DensityUnits=kg/m^3  DensityUse=false  GraphicsMode=GFXFILE  GraphicsFileName=Ensamblaje1 - brazo1fribracarbono-2.STL  BodyColorSelMode=COLORPALETTE  BodyColor=[0.16863 0.50588 0.33726]  AttachedToCS=CS1  CG=Right$CG$[-0.00476641 0.271763 0.269142]$WORLD$WORLD$m$[0 -1 0;0.929227 0 -0.36951;0.36951 0 0.929227]$3x3 Transform$rad$WORLD$false$brazo1fribracarbono-2::CG(AUTOGEN)  WorkingFrames=Right$CS1$[-0.00428141 0.198979 0.253651]$WORLD$WORLD$m$[0 -1 0;0.929227 0 -0.36951;0.36951 0 0.929227]$3x3 Transform$rad$WORLD$false$brazo1fribracarbono-2::CS1(AUTOGEN)#Right$CS2$[-0.00525141 0.317724 0.296028]$WORLD$WORLD$m$[1 0 0;0 1 0;0 0 1]$3x3 Transform$rad$WORLD$false$Copia de motordymaxixel^Ensamblaje1-2:-:brazo1fribracarbono-2::brazo1fribracarbono-2(AUTOGEN)#Right$CS3$[-0.00428141 0.198979 0.253651]$WORLD$WORLD$m$[1 0 0;0 1 0;0 0 1]$3x3 Transform$rad$WORLD$true$brazo1fribracarbono-2:-:soporteM (1)-2::brazo1fribracarbono-2(AUTOGEN)#Right$CS4$[-0.00428141 0.198979 0.253651]$WORLD$WORLD$m$[1 0 0;0 1 0;0 0 1]$3x3 Transform$rad$WORLD$true$aumento-1:-:brazo1fribracarbono-2::brazo1fribracarbono-2(AUTOGEN)#Left$CS5$[-0.00525141 0.269172 0.276721]$WORLD$WORLD$m$[1 0 0;0 1 0;0 0 1]$3x3 Transform$rad$WORLD$true$brazo1fribracarbono-2:-:soporteM (1)-1::brazo1fribracarbono-2(AUTOGEN)#Left$CS6$[-0.00428141 0.198979 0.253651]$WORLD$WORLD$m$[1 0 0;0 1 0;0 0 1]$3x3 Transform$rad$WORLD$true$bacedymamixel-1:-:brazo1fribracarbono-2::brazo1fribracarbono-2(AUTOGEN)  CGPos=[-0.00476641 0.271763 0.269142]  CGRot=[0 -1 0;0.929227 0 -0.36951;0.36951 0 0.929227]  CS0Pos=[]  CS0Rot=[]  CS1Pos=[-0.00428141 0.198979 0.253651]  CS1Rot=[0 -1 0;0.929227 0 -0.36951;0.36951 0 0.929227]  CS2Pos=[-0.00525141 0.317724 0.296028]  CS2Rot=[1 0 0;0 1 0;0 0 1]  CS3Pos=[-0.00428141 0.198979 0.253651]  CS3Rot=[1 0 0;0 1 0;0 0 1]  CS4Pos=[-0.00428141 0.198979 0.253651]  CS4Rot=[1 0 0;0 1 0;0 0 1]  CS5Pos=[-0.00525141 0.269172 0.276721]  CS5Rot=[1 0 0;0 1 0;0 0 1]  CS6Pos=[-0.00428141 0.198979 0.253651]  CS6Rot=[1 0 0;0 1 0;0 0 1]  CS7Pos=[]  CS7Rot=[]  CS8Pos=[]  CS8Rot=[]  CS9Pos=[]  CS9Rot=[]  CS10Pos=[]  CS10Rot=[]  CS11Pos=[]  CS11Rot=[]  CS12Pos=[]  CS12Rot=[]  CS13Pos=[]  CS13Rot=[]  CS14Pos=[]  CS14Rot=[]  CS15Pos=[]  CS15Rot=[]  CS16Pos=[]  CS16Rot=[]  CS17Pos=[]  CS17Rot=[]  CS18Pos=[]  CS18Rot=[]  CS19Pos=[]  CS19Rot=[]  CS20Pos=[]  CS20Rot=[]
  brazo2frubra-1 : mblibv1/Bodies/Body  LConnTagsString=CS2|CS3  UpdateFromCAD=on  PMImportedID=brazo2frubra-1  DialogClass=MechanicalBodyBlock  Mass=0.00552755  MassUnits=kg  InertiaUnits=kg*m^2  Inertia=[4.47123e-07,0,0;0,5.58282e-06,0;0,0,5.13656e-06]  Shape=Cylinder  ShapeDims=[1 1]  ShapeUnits=m  ShapeUse=false  Density=1  DensityUnits=kg/m^3  DensityUse=false  GraphicsMode=GFXFILE  GraphicsFileName=Ensamblaje1 - brazo2frubra-1.STL  BodyColorSelMode=COLORPALETTE  BodyColor=[1;1;0]  AttachedToCS=CS1  CG=Right$CG$[-0.00576641 0.375331 0.267077]$WORLD$WORLD$m$[0 1 0;0.520016 0 -0.854156;-0.854156 0 -0.520016]$3x3 Transform$rad$WORLD$false$brazo2frubra-1::CG(AUTOGEN)  WorkingFrames=Right$CS1$[-0.00625141 0.337216 0.305646]$WORLD$WORLD$m$[0 1 0;0.520016 0 -0.854156;-0.854156 0 -0.520016]$3x3 Transform$rad$WORLD$false$brazo2frubra-1::CS1(AUTOGEN)#Left$CS2$[-0.00528141 0.358569 0.318647]$WORLD$WORLD$m$[1 0 0;0 1 0;0 0 1]$3x3 Transform$rad$WORLD$true$bacedymamixel-2:-:brazo2frubra-1::brazo2frubra-1(AUTOGEN)#Left$CS3$[-0.00528141 0.389941 0.227696]$WORLD$WORLD$m$[1 0 0;0 1 0;0 0 1]$3x3 Transform$rad$WORLD$true$brazo2frubra-1:-:soporte-3::brazo2frubra-1(AUTOGEN)  CGPos=[-0.00576641 0.375331 0.267077]  CGRot=[0 1 0;0.520016 0 -0.854156;-0.854156 0 -0.520016]  CS0Pos=[]  CS0Rot=[]  CS1Pos=[-0.00625141 0.337216 0.305646]  CS1Rot=[0 1 0;0.520016 0 -0.854156;-0.854156 0 -0.520016]  CS2Pos=[-0.00528141 0.358569 0.318647]  CS2Rot=[1 0 0;0 1 0;0 0 1]  CS3Pos=[-0.00528141 0.389941 0.227696]  CS3Rot=[1 0 0;0 1 0;0 0 1]  CS4Pos=[]  CS4Rot=[]  CS5Pos=[]  CS5Rot=[]  CS6Pos=[]  CS6Rot=[]  CS7Pos=[]  CS7Rot=[]  CS8Pos=[]  CS8Rot=[]  CS9Pos=[]  CS9Rot=[]  CS10Pos=[]  CS10Rot=[]  CS11Pos=[]  CS11Rot=[]  CS12Pos=[]  CS12Rot=[]  CS13Pos=[]  CS13Rot=[]  CS14Pos=[]  CS14Rot=[]  CS15Pos=[]  CS15Rot=[]  CS16Pos=[]  CS16Rot=[]  CS17Pos=[]  CS17Rot=[]  CS18Pos=[]  CS18Rot=[]  CS19Pos=[]  CS19Rot=[]  CS20Pos=[]  CS20Rot=[]
  brazo2frubra-2 : mblibv1/Bodies/Body  LConnTagsString=CS2  UpdateFromCAD=on  PMImportedID=brazo2frubra-2  DialogClass=MechanicalBodyBlock  Mass=0.00552755  MassUnits=kg  InertiaUnits=kg*m^2  Inertia=[4.47123e-07,0,0;0,5.58282e-06,0;0,0,5.13656e-06]  Shape=Cylinder  ShapeDims=[1 1]  ShapeUnits=m  ShapeUse=false  Density=1  DensityUnits=kg/m^3  DensityUse=false  GraphicsMode=GFXFILE  GraphicsFileName=Ensamblaje1 - brazo2frubra-2.STL  BodyColorSelMode=COLORPALETTE  BodyColor=[0.74902;0.74902;0]  AttachedToCS=CS1  CG=Right$CG$[0.0432036 0.375331 0.267077]$WORLD$WORLD$m$[0 -1 0;0.520016 0 0.854156;-0.854156 0 0.520016]$3x3 Transform$rad$WORLD$false$brazo2frubra-2::CG(AUTOGEN)  WorkingFrames=Right$CS1$[0.0436886 0.358569 0.318647]$WORLD$WORLD$m$[0 -1 0;0.520016 0 0.854156;-0.854156 0 0.520016]$3x3 Transform$rad$WORLD$false$brazo2frubra-2::CS1(AUTOGEN)#Left$CS2$[0.0427186 0.37781 0.287043]$WORLD$WORLD$m$[1 0 0;0 1 0;0 0 1]$3x3 Transform$rad$WORLD$true$bacedymamixel-2:-:brazo2frubra-2::brazo2frubra-2(AUTOGEN)  CGPos=[0.0432036 0.375331 0.267077]  CGRot=[0 -1 0;0.520016 0 0.854156;-0.854156 0 0.520016]  CS0Pos=[]  CS0Rot=[]  CS1Pos=[0.0436886 0.358569 0.318647]  CS1Rot=[0 -1 0;0.520016 0 0.854156;-0.854156 0 0.520016]  CS2Pos=[0.0427186 0.37781 0.287043]  CS2Rot=[1 0 0;0 1 0;0 0 1]  CS3Pos=[]  CS3Rot=[]  CS4Pos=[]  CS4Rot=[]  CS5Pos=[]  CS5Rot=[]  CS6Pos=[]  CS6Rot=[]  CS7Pos=[]  CS7Rot=[]  CS8Pos=[]  CS8Rot=[]  CS9Pos=[]  CS9Rot=[]  CS10Pos=[]  CS10Rot=[]  CS11Pos=[]  CS11Rot=[]  CS12Pos=[]  CS12Rot=[]  CS13Pos=[]  CS13Rot=[]  CS14Pos=[]  CS14Rot=[]  CS15Pos=[]  CS15Rot=[]  CS16Pos=[]  CS16Rot=[]  CS17Pos=[]  CS17Rot=[]  CS18Pos=[]  CS18Rot=[]  CS19Pos=[]  CS19Rot=[]  CS20Pos=[]  CS20Rot=[]
  motor 1dynamixel-1 : mblibv1/Bodies/Body  LConnTagsString=CS2  RConnTagsString=CS1|CS3  UpdateFromCAD=on  PMImportedID=motor 1dynamixel-1  DialogClass=MechanicalBodyBlock  Mass=0.00144762  MassUnits=kg  InertiaUnits=kg*m^2  Inertia=[1.88829e-07,0,0;0,1.88829e-07,0;0,0,6.4082e-09]  Shape=Cylinder  ShapeDims=[1 1]  ShapeUnits=m  ShapeUse=false  Density=1  DensityUnits=kg/m^3  DensityUse=false  GraphicsMode=GFXFILE  GraphicsFileName=Ensamblaje1 - motor 1dynamixel-1.STL  BodyColorSelMode=COLORPALETTE  BodyColor=[1 1 0]  AttachedToCS=CS1  CG=Right$CG$[0.0192847 0.214749 0.24647]$WORLD$WORLD$m$[0 0 1;0 1 0;-1 0 0]$3x3 Transform$rad$WORLD$false$motor 1dynamixel-1::CG(AUTOGEN)  WorkingFrames=Right$CS1$[-0.00028141 0.214749 0.24647]$WORLD$WORLD$m$[0 0 1;0 1 0;-1 0 0]$3x3 Transform$rad$WORLD$true$motor 1dynamixel-1::CS1(AUTOGEN)#Left$CS2$[0.0367186 0.214749 0.24647]$WORLD$WORLD$m$[1 0 0;0 1 0;0 0 1]$3x3 Transform$rad$WORLD$true$Copia de motordymaxixel^Ensamblaje1-1:-:motor 1dynamixel-1::motor 1dynamixel-1(AUTOGEN)#Right$CS3$[-0.00028141 0.214749 0.24647]$WORLD$WORLD$m$[1 0 0;0 1 0;0 0 1]$3x3 Transform$rad$WORLD$true$motor 1dynamixel-1:-:motordymamixel-1::motor 1dynamixel-1(AUTOGEN)  CGPos=[0.0192847 0.214749 0.24647]  CGRot=[0 0 1;0 1 0;-1 0 0]  CS0Pos=[]  CS0Rot=[]  CS1Pos=[-0.00028141 0.214749 0.24647]  CS1Rot=[0 0 1;0 1 0;-1 0 0]  CS2Pos=[0.0367186 0.214749 0.24647]  CS2Rot=[1 0 0;0 1 0;0 0 1]  CS3Pos=[-0.00028141 0.214749 0.24647]  CS3Rot=[1 0 0;0 1 0;0 0 1]  CS4Pos=[]  CS4Rot=[]  CS5Pos=[]  CS5Rot=[]  CS6Pos=[]  CS6Rot=[]  CS7Pos=[]  CS7Rot=[]  CS8Pos=[]  CS8Rot=[]  CS9Pos=[]  CS9Rot=[]  CS10Pos=[]  CS10Rot=[]  CS11Pos=[]  CS11Rot=[]  CS12Pos=[]  CS12Rot=[]  CS13Pos=[]  CS13Rot=[]  CS14Pos=[]  CS14Rot=[]  CS15Pos=[]  CS15Rot=[]  CS16Pos=[]  CS16Rot=[]  CS17Pos=[]  CS17Rot=[]  CS18Pos=[]  CS18Rot=[]  CS19Pos=[]  CS19Rot=[]  CS20Pos=[]  CS20Rot=[]
  motor 1dynamixel-2 : mblibv1/Bodies/Body  RConnTagsString=CS2|CS3  UpdateFromCAD=on  PMImportedID=motor 1dynamixel-2  DialogClass=MechanicalBodyBlock  Mass=0.00144762  MassUnits=kg  InertiaUnits=kg*m^2  Inertia=[1.88829e-07,0,0;0,1.88829e-07,0;0,0,6.4082e-09]  Shape=Cylinder  ShapeDims=[1 1]  ShapeUnits=m  ShapeUse=false  Density=1  DensityUnits=kg/m^3  DensityUse=false  GraphicsMode=GFXFILE  GraphicsFileName=Ensamblaje1 - motor 1dynamixel-2.STL  BodyColorSelMode=COLORPALETTE  BodyColor=[1;1;0]  AttachedToCS=CS1  CG=Right$CG$[0.0182847 0.354133 0.301897]$WORLD$WORLD$m$[0 0 1;0.0682213 -0.99767 0;0.99767 0.0682213 0]$3x3 Transform$rad$WORLD$false$motor 1dynamixel-2::CG(AUTOGEN)  WorkingFrames=Right$CS1$[-0.00128141 0.354133 0.301897]$WORLD$WORLD$m$[0 0 1;0.0682213 -0.99767 0;0.99767 0.0682213 0]$3x3 Transform$rad$WORLD$false$motor 1dynamixel-2::CS1(AUTOGEN)#Right$CS2$[-0.00128141 0.354133 0.301897]$WORLD$WORLD$m$[1 0 0;0 1 0;0 0 1]$3x3 Transform$rad$WORLD$true$motor 1dynamixel-2:-:motordymamixel-2::motor 1dynamixel-2(AUTOGEN)#Right$CS3$[0.0357186 0.354133 0.301897]$WORLD$WORLD$m$[1 0 0;0 1 0;0 0 1]$3x3 Transform$rad$WORLD$true$Copia de motordymaxixel^Ensamblaje1-2:-:motor 1dynamixel-2::motor 1dynamixel-2(AUTOGEN)  CGPos=[0.0182847 0.354133 0.301897]  CGRot=[0 0 1;0.0682213 -0.99767 0;0.99767 0.0682213 0]  CS0Pos=[]  CS0Rot=[]  CS1Pos=[-0.00128141 0.354133 0.301897]  CS1Rot=[0 0 1;0.0682213 -0.99767 0;0.99767 0.0682213 0]  CS2Pos=[-0.00128141 0.354133 0.301897]  CS2Rot=[1 0 0;0 1 0;0 0 1]  CS3Pos=[0.0357186 0.354133 0.301897]  CS3Rot=[1 0 0;0 1 0;0 0 1]  CS4Pos=[]  CS4Rot=[]  CS5Pos=[]  CS5Rot=[]  CS6Pos=[]  CS6Rot=[]  CS7Pos=[]  CS7Rot=[]  CS8Pos=[]  CS8Rot=[]  CS9Pos=[]  CS9Rot=[]  CS10Pos=[]  CS10Rot=[]  CS11Pos=[]  CS11Rot=[]  CS12Pos=[]  CS12Rot=[]  CS13Pos=[]  CS13Rot=[]  CS14Pos=[]  CS14Rot=[]  CS15Pos=[]  CS15Rot=[]  CS16Pos=[]  CS16Rot=[]  CS17Pos=[]  CS17Rot=[]  CS18Pos=[]  CS18Rot=[]  CS19Pos=[]  CS19Rot=[]  CS20Pos=[]  CS20Rot=[]
  motordymamixel-1 : mblibv1/Bodies/Body  LConnTagsString=CS2  UpdateFromCAD=on  PMImportedID=motordymamixel-1  DialogClass=MechanicalBodyBlock  Mass=0.00230392  MassUnits=kg  InertiaUnits=kg*m^2  Inertia=[7.81038e-08,-1.705e-14,0;-1.705e-14,7.7877e-08,0;0,0,1.49837e-07]  Shape=Cylinder  ShapeDims=[1 1]  ShapeUnits=m  ShapeUse=false  Density=1  DensityUnits=kg/m^3  DensityUse=false  GraphicsMode=GFXFILE  GraphicsFileName=Ensamblaje1 - motordymamixel-1.STL  BodyColorSelMode=COLORPALETTE  BodyColor=[0.078431 0.16863 0.54902]  AttachedToCS=CS1  CG=Right$CG$[0.00171859 0.214744 0.24647]$WORLD$WORLD$m$[0 0 -1;-0.265315 0.964162 0;0.964162 0.265315 0]$3x3 Transform$rad$WORLD$false$motordymamixel-1::CG(AUTOGEN)  WorkingFrames=Right$CS1$[0.00371859 0.214749 0.24647]$WORLD$WORLD$m$[0 0 -1;-0.265315 0.964162 0;0.964162 0.265315 0]$3x3 Transform$rad$WORLD$false$motordymamixel-1::CS1(AUTOGEN)#Left$CS2$[-0.00028141 0.214749 0.24647]$WORLD$WORLD$m$[1 0 0;0 1 0;0 0 1]$3x3 Transform$rad$WORLD$true$motor 1dynamixel-1:-:motordymamixel-1::motordymamixel-1(AUTOGEN)#Left$CS3$[-0.00028141 0.214749 0.24647]$WORLD$WORLD$m$[1 0 0;0 1 0;0 0 1]$3x3 Transform$rad$WORLD$false$bacedymamixel-1:-:motordymamixel-1::motordymamixel-1(AUTOGEN)  CGPos=[0.00171859 0.214744 0.24647]  CGRot=[0 0 -1;-0.265315 0.964162 0;0.964162 0.265315 0]  CS0Pos=[]  CS0Rot=[]  CS1Pos=[0.00371859 0.214749 0.24647]  CS1Rot=[0 0 -1;-0.265315 0.964162 0;0.964162 0.265315 0]  CS2Pos=[-0.00028141 0.214749 0.24647]  CS2Rot=[1 0 0;0 1 0;0 0 1]  CS3Pos=[-0.00028141 0.214749 0.24647]  CS3Rot=[1 0 0;0 1 0;0 0 1]  CS4Pos=[]  CS4Rot=[]  CS5Pos=[]  CS5Rot=[]  CS6Pos=[]  CS6Rot=[]  CS7Pos=[]  CS7Rot=[]  CS8Pos=[]  CS8Rot=[]  CS9Pos=[]  CS9Rot=[]  CS10Pos=[]  CS10Rot=[]  CS11Pos=[]  CS11Rot=[]  CS12Pos=[]  CS12Rot=[]  CS13Pos=[]  CS13Rot=[]  CS14Pos=[]  CS14Rot=[]  CS15Pos=[]  CS15Rot=[]  CS16Pos=[]  CS16Rot=[]  CS17Pos=[]  CS17Rot=[]  CS18Pos=[]  CS18Rot=[]  CS19Pos=[]  CS19Rot=[]  CS20Pos=[]  CS20Rot=[]
  motordymamixel-2 : mblibv1/Bodies/Body  LConnTagsString=CS2|CS3  UpdateFromCAD=on  PMImportedID=motordymamixel-2  DialogClass=MechanicalBodyBlock  Mass=0.00230392  MassUnits=kg  InertiaUnits=kg*m^2  Inertia=[7.81038e-08,-1.705e-14,0;-1.705e-14,7.7877e-08,0;0,0,1.49837e-07]  Shape=Cylinder  ShapeDims=[1 1]  ShapeUnits=m  ShapeUse=false  Density=1  DensityUnits=kg/m^3  DensityUse=false  GraphicsMode=GFXFILE  GraphicsFileName=Ensamblaje1 - motordymamixel-2.STL  BodyColorSelMode=COLORPALETTE  BodyColor=[0.078431 0.16863 0.54902]  AttachedToCS=CS1  CG=Right$CG$[0.00071859 0.354128 0.301898]$WORLD$WORLD$m$[0 0 -1;0 1 0;1 0 0]$3x3 Transform$rad$WORLD$false$motordymamixel-2::CG(AUTOGEN)  WorkingFrames=Right$CS1$[0.00271859 0.354133 0.301897]$WORLD$WORLD$m$[0 0 -1;0 1 0;1 0 0]$3x3 Transform$rad$WORLD$false$motordymamixel-2::CS1(AUTOGEN)#Left$CS2$[-0.00128141 0.354133 0.301897]$WORLD$WORLD$m$[1 0 0;0 1 0;0 0 1]$3x3 Transform$rad$WORLD$true$bacedymamixel-2:-:motordymamixel-2::motordymamixel-2(AUTOGEN)#Left$CS3$[-0.00128141 0.354133 0.301897]$WORLD$WORLD$m$[1 0 0;0 1 0;0 0 1]$3x3 Transform$rad$WORLD$true$motor 1dynamixel-2:-:motordymamixel-2::motordymamixel-2(AUTOGEN)  CGPos=[0.00071859 0.354128 0.301898]  CGRot=[0 0 -1;0 1 0;1 0 0]  CS0Pos=[]  CS0Rot=[]  CS1Pos=[0.00271859 0.354133 0.301897]  CS1Rot=[0 0 -1;0 1 0;1 0 0]  CS2Pos=[-0.00128141 0.354133 0.301897]  CS2Rot=[1 0 0;0 1 0;0 0 1]  CS3Pos=[-0.00128141 0.354133 0.301897]  CS3Rot=[1 0 0;0 1 0;0 0 1]  CS4Pos=[]  CS4Rot=[]  CS5Pos=[]  CS5Rot=[]  CS6Pos=[]  CS6Rot=[]  CS7Pos=[]  CS7Rot=[]  CS8Pos=[]  CS8Rot=[]  CS9Pos=[]  CS9Rot=[]  CS10Pos=[]  CS10Rot=[]  CS11Pos=[]  CS11Rot=[]  CS12Pos=[]  CS12Rot=[]  CS13Pos=[]  CS13Rot=[]  CS14Pos=[]  CS14Rot=[]  CS15Pos=[]  CS15Rot=[]  CS16Pos=[]  CS16Rot=[]  CS17Pos=[]  CS17Rot=[]  CS18Pos=[]  CS18Rot=[]  CS19Pos=[]  CS19Rot=[]  CS20Pos=[]  CS20Rot=[]
  par-1 : mblibv1/Bodies/Body  LConnTagsString=CS2  RConnTagsString=CS3  UpdateFromCAD=on  PMImportedID=par-1  DialogClass=MechanicalBodyBlock  Mass=0.0892915  MassUnits=kg  InertiaUnits=kg*m^2  Inertia=[0.00017021,1.37311e-08,0;1.37311e-08,0.000143513,0;0,0,0.000313589]  Shape=Cylinder  ShapeDims=[1 1]  ShapeUnits=m  ShapeUse=false  Density=1  DensityUnits=kg/m^3  DensityUse=false  GraphicsMode=GFXFILE  GraphicsFileName=Ensamblaje1 - par-1.STL  BodyColorSelMode=COLORPALETTE  BodyColor=[0;1;1]  AttachedToCS=CS1  CG=Right$CG$[0.0217437 0.176811 0.202]$WORLD$WORLD$m$[1 0 0;0 1 0;0 0 1]$3x3 Transform$rad$WORLD$false$par-1::CG(AUTOGEN)  WorkingFrames=Right$CS1$[-0.0662814 0.0727487 0.2005]$WORLD$WORLD$m$[1 0 0;0 1 0;0 0 1]$3x3 Transform$rad$WORLD$false$par-1::CS1(AUTOGEN)#Left$CS2$[0.0217437 0.176811 0.202]$WORLD$WORLD$m$[1 0 0;0 1 0;0 0 1]$3x3 Transform$rad$WORLD$true$Ensamblaje1/RootPart:-:par-1::par-1(AUTOGEN)#Right$CS3$[-0.0342814 0.200749 0.2035]$WORLD$WORLD$m$[1 0 0;0 1 0;0 0 1]$3x3 Transform$rad$WORLD$true$Pieza1bASE-1:-:par-1::par-1(AUTOGEN)  CGPos=[0.0217437 0.176811 0.202]  CGRot=[1 0 0;0 1 0;0 0 1]  CS0Pos=[]  CS0Rot=[]  CS1Pos=[-0.0662814 0.0727487 0.2005]  CS1Rot=[1 0 0;0 1 0;0 0 1]  CS2Pos=[0.0217437 0.176811 0.202]  CS2Rot=[1 0 0;0 1 0;0 0 1]  CS3Pos=[-0.0342814 0.200749 0.2035]  CS3Rot=[1 0 0;0 1 0;0 0 1]  CS4Pos=[]  CS4Rot=[]  CS5Pos=[]  CS5Rot=[]  CS6Pos=[]  CS6Rot=[]  CS7Pos=[]  CS7Rot=[]  CS8Pos=[]  CS8Rot=[]  CS9Pos=[]  CS9Rot=[]  CS10Pos=[]  CS10Rot=[]  CS11Pos=[]  CS11Rot=[]  CS12Pos=[]  CS12Rot=[]  CS13Pos=[]  CS13Rot=[]  CS14Pos=[]  CS14Rot=[]  CS15Pos=[]  CS15Rot=[]  CS16Pos=[]  CS16Rot=[]  CS17Pos=[]  CS17Rot=[]  CS18Pos=[]  CS18Rot=[]  CS19Pos=[]  CS19Rot=[]  CS20Pos=[]  CS20Rot=[]
  soporte-3 : mblibv1/Bodies/Body  RConnTagsString=CS2  UpdateFromCAD=on  PMImportedID=soporte-3  DialogClass=MechanicalBodyBlock  Mass=0.0046869  MassUnits=kg  InertiaUnits=kg*m^2  Inertia=[3.24537e-07,0,0;0,1.47562e-06,0;0,0,1.20985e-06]  Shape=Cylinder  ShapeDims=[1 1]  ShapeUnits=m  ShapeUse=false  Density=1  DensityUnits=kg/m^3  DensityUse=false  GraphicsMode=GFXFILE  GraphicsFileName=Ensamblaje1 - soporte-3.STL  BodyColorSelMode=COLORPALETTE  BodyColor=[0;0;1]  AttachedToCS=CS1  CG=Right$CG$[0.0187186 0.399419 0.227512]$WORLD$WORLD$m$[1 0 0;0 0.520016 0.854156;0 -0.854156 0.520016]$3x3 Transform$rad$WORLD$false$soporte-3::CG(AUTOGEN)  WorkingFrames=Right$CS1$[-0.00528141 0.384017 0.228772]$WORLD$WORLD$m$[1 0 0;0 0.520016 0.854156;0 -0.854156 0.520016]$3x3 Transform$rad$WORLD$false$soporte-3::CS1(AUTOGEN)#Right$CS2$[-0.00528141 0.389941 0.227696]$WORLD$WORLD$m$[1 0 0;0 1 0;0 0 1]$3x3 Transform$rad$WORLD$true$brazo2frubra-1:-:soporte-3::soporte-3(AUTOGEN)  CGPos=[0.0187186 0.399419 0.227512]  CGRot=[1 0 0;0 0.520016 0.854156;0 -0.854156 0.520016]  CS0Pos=[]  CS0Rot=[]  CS1Pos=[-0.00528141 0.384017 0.228772]  CS1Rot=[1 0 0;0 0.520016 0.854156;0 -0.854156 0.520016]  CS2Pos=[-0.00528141 0.389941 0.227696]  CS2Rot=[1 0 0;0 1 0;0 0 1]  CS3Pos=[]  CS3Rot=[]  CS4Pos=[]  CS4Rot=[]  CS5Pos=[]  CS5Rot=[]  CS6Pos=[]  CS6Rot=[]  CS7Pos=[]  CS7Rot=[]  CS8Pos=[]  CS8Rot=[]  CS9Pos=[]  CS9Rot=[]  CS10Pos=[]  CS10Rot=[]  CS11Pos=[]  CS11Rot=[]  CS12Pos=[]  CS12Rot=[]  CS13Pos=[]  CS13Rot=[]  CS14Pos=[]  CS14Rot=[]  CS15Pos=[]  CS15Rot=[]  CS16Pos=[]  CS16Rot=[]  CS17Pos=[]  CS17Rot=[]  CS18Pos=[]  CS18Rot=[]  CS19Pos=[]  CS19Rot=[]  CS20Pos=[]  CS20Rot=[]
  soporteM (1)-1 : mblibv1/Bodies/Body  LConnTagsString=CS2|CS3  UpdateFromCAD=on  PMImportedID=soporteM (1)-1  DialogClass=MechanicalBodyBlock  Mass=0.00200267  MassUnits=kg  InertiaUnits=kg*m^2  Inertia=[3.45021e-08,0,0;0,6.27654e-07,0;0,0,6.19915e-07]  Shape=Cylinder  ShapeDims=[1 1]  ShapeUnits=m  ShapeUse=false  Density=1  DensityUnits=kg/m^3  DensityUse=false  GraphicsMode=GFXFILE  GraphicsFileName=Ensamblaje1 - soporteM (1)-1.STL  BodyColorSelMode=COLORPALETTE  BodyColor=[0 0.6 0.6]  AttachedToCS=CS1  CG=Right$CG$[0.0197186 0.264891 0.275019]$WORLD$WORLD$m$[1 0 0;0 0.36951 0.929227;0 -0.929227 0.36951]$3x3 Transform$rad$WORLD$false$soporteM (1)-1::CG(AUTOGEN)  WorkingFrames=Right$CS1$[-0.00428141 0.261934 0.278686]$WORLD$WORLD$m$[1 0 0;0 0.36951 0.929227;0 -0.929227 0.36951]$3x3 Transform$rad$WORLD$false$soporteM (1)-1::CS1(AUTOGEN)#Left$CS2$[0.0437186 0.208217 0.230421]$WORLD$WORLD$m$[1 0 0;0 1 0;0 0 1]$3x3 Transform$rad$WORLD$true$brazo1fribracarbono-1:-:soporteM (1)-1::soporteM (1)-1(AUTOGEN)#Left$CS3$[-0.00428141 0.269172 0.276721]$WORLD$WORLD$m$[1 0 0;0 1 0;0 0 1]$3x3 Transform$rad$WORLD$true$brazo1fribracarbono-2:-:soporteM (1)-1::soporteM (1)-1(AUTOGEN)  CGPos=[0.0197186 0.264891 0.275019]  CGRot=[1 0 0;0 0.36951 0.929227;0 -0.929227 0.36951]  CS0Pos=[]  CS0Rot=[]  CS1Pos=[-0.00428141 0.261934 0.278686]  CS1Rot=[1 0 0;0 0.36951 0.929227;0 -0.929227 0.36951]  CS2Pos=[0.0437186 0.208217 0.230421]  CS2Rot=[1 0 0;0 1 0;0 0 1]  CS3Pos=[-0.00428141 0.269172 0.276721]  CS3Rot=[1 0 0;0 1 0;0 0 1]  CS4Pos=[]  CS4Rot=[]  CS5Pos=[]  CS5Rot=[]  CS6Pos=[]  CS6Rot=[]  CS7Pos=[]  CS7Rot=[]  CS8Pos=[]  CS8Rot=[]  CS9Pos=[]  CS9Rot=[]  CS10Pos=[]  CS10Rot=[]  CS11Pos=[]  CS11Rot=[]  CS12Pos=[]  CS12Rot=[]  CS13Pos=[]  CS13Rot=[]  CS14Pos=[]  CS14Rot=[]  CS15Pos=[]  CS15Rot=[]  CS16Pos=[]  CS16Rot=[]  CS17Pos=[]  CS17Rot=[]  CS18Pos=[]  CS18Rot=[]  CS19Pos=[]  CS19Rot=[]  CS20Pos=[]  CS20Rot=[]
  soporteM (1)-2 : mblibv1/Bodies/Body  LConnTagsString=CS2|CS3  UpdateFromCAD=on  PMImportedID=soporteM (1)-2  DialogClass=MechanicalBodyBlock  Mass=0.00200267  MassUnits=kg  InertiaUnits=kg*m^2  Inertia=[3.45021e-08,0,0;0,6.27654e-07,0;0,0,6.19915e-07]  Shape=Cylinder  ShapeDims=[1 1]  ShapeUnits=m  ShapeUse=false  Density=1  DensityUnits=kg/m^3  DensityUse=false  GraphicsMode=GFXFILE  GraphicsFileName=Ensamblaje1 - soporteM (1)-2.STL  BodyColorSelMode=COLORPALETTE  BodyColor=[0.0431373;0.517647;0.780392]  AttachedToCS=CS1  CG=Right$CG$[0.0197186 0.270803 0.260151]$WORLD$WORLD$m$[1 0 0;0 0.36951 0.929227;0 -0.929227 0.36951]$3x3 Transform$rad$WORLD$false$soporteM (1)-2::CG(AUTOGEN)  WorkingFrames=Right$CS1$[-0.00428141 0.267846 0.263818]$WORLD$WORLD$m$[1 0 0;0 0.36951 0.929227;0 -0.929227 0.36951]$3x3 Transform$rad$WORLD$false$soporteM (1)-2::CS1(AUTOGEN)#Left$CS2$[0.0407186 0.275085 0.261853]$WORLD$WORLD$m$[1 0 0;0 1 0;0 0 1]$3x3 Transform$rad$WORLD$true$brazo1fribracarbono-1:-:soporteM (1)-2::soporteM (1)-2(AUTOGEN)#Left$CS3$[-0.00428141 0.198979 0.253651]$WORLD$WORLD$m$[1 0 0;0 1 0;0 0 1]$3x3 Transform$rad$WORLD$true$brazo1fribracarbono-2:-:soporteM (1)-2::soporteM (1)-2(AUTOGEN)  CGPos=[0.0197186 0.270803 0.260151]  CGRot=[1 0 0;0 0.36951 0.929227;0 -0.929227 0.36951]  CS0Pos=[]  CS0Rot=[]  CS1Pos=[-0.00428141 0.267846 0.263818]  CS1Rot=[1 0 0;0 0.36951 0.929227;0 -0.929227 0.36951]  CS2Pos=[0.0407186 0.275085 0.261853]  CS2Rot=[1 0 0;0 1 0;0 0 1]  CS3Pos=[-0.00428141 0.198979 0.253651]  CS3Rot=[1 0 0;0 1 0;0 0 1]  CS4Pos=[]  CS4Rot=[]  CS5Pos=[]  CS5Rot=[]  CS6Pos=[]  CS6Rot=[]  CS7Pos=[]  CS7Rot=[]  CS8Pos=[]  CS8Rot=[]  CS9Pos=[]  CS9Rot=[]  CS10Pos=[]  CS10Rot=[]  CS11Pos=[]  CS11Rot=[]  CS12Pos=[]  CS12Rot=[]  CS13Pos=[]  CS13Rot=[]  CS14Pos=[]  CS14Rot=[]  CS15Pos=[]  CS15Rot=[]  CS16Pos=[]  CS16Rot=[]  CS17Pos=[]  CS17Rot=[]  CS18Pos=[]  CS18Rot=[]  CS19Pos=[]  CS19Rot=[]  CS20Pos=[]  CS20Rot=[]
  connections:
  RootPart/RConn1 -- Weld/LConn1
  Weld/RConn1 -- Pieza1bASE-1/LConn1
  RootPart/RConn2 -- Weld1/LConn1
  Weld1/RConn1 -- par-1/LConn1
  bacedymamixel-2/RConn1 -- Revolute/LConn1
  Revolute/RConn1 -- motordymamixel-2/LConn1
  motor 1dynamixel-2/RConn1 -- Revolute1/LConn1
  Revolute1/RConn1 -- motordymamixel-2/LConn2
  bacedymamixel-2/RConn2 -- Weld2/LConn1
  Weld2/RConn1 -- brazo2frubra-1/LConn1
  bacedymamixel-2/RConn3 -- Weld3/LConn1
  Weld3/RConn1 -- brazo2frubra-2/LConn1
  soporte-3/RConn1 -- Weld5/LConn1
  Weld5/RConn1 -- brazo2frubra-1/LConn2
  motor 1dynamixel-2/RConn2 -- Revolute2/LConn1
  Weld19/RConn1 -- Copia de motordymaxixel^Ensamblaje1-2/LConn2
  Weld13/LConn1 -- brazo1fribracarbono-2/RConn1
  brazo1fribracarbono-1/RConn2 -- Weld14/LConn1
  soporteM (1)-1/LConn1 -- Weld14/RConn1
  soporteM (1)-1/LConn2 -- Weld16/RConn1
  Copia de motordymaxixel^Ensamblaje1-1/RConn1 -- Weld7/LConn1
  Weld7/RConn1 -- bacedymami-1/LConn1
  Pieza1bASE-1/RConn1 -- Weld8/LConn1
  Weld8/RConn1 -- bacedymami-1/LConn2
  bacedymamixel-1/RConn1 -- Weld9/LConn1
  Weld9/RConn1 -- brazo1fribracarbono-1/LConn2
  bacedymamixel-1/RConn2 -- Weld10/LConn1
  Weld10/RConn1 -- brazo1fribracarbono-2/LConn2
  RootGround/RConn1 -- Weld11/LConn1
  Weld11/RConn1 -- RootPart/LConn1
  RootGround/LConn1 -- Machine Environment/RConn1
  Weld12/LConn1 -- par-1/RConn1
  Weld12/RConn1 -- Pieza1bASE-1/LConn2
  Weld13/RConn1 -- soporteM (1)-2/LConn2
  Copia de motordymaxixel^Ensamblaje1-1/LConn1 -- Revolute3/LConn1
  Weld17/RConn1 -- motordymamixel-1/LConn1
  Weld17/LConn1 -- motor 1dynamixel-1/RConn1
  Weld18/LConn1 -- motor 1dynamixel-1/RConn2
  motor 1dynamixel-1/LConn1 -- Revolute3/RConn1
  soporteM (1)-2/LConn1 -- Weld15/RConn1
  Weld15/LConn1 -- brazo1fribracarbono-1/LConn1
  Weld16/LConn1 -- brazo1fribracarbono-2/LConn1
  Weld18/RConn1 -- bacedymamixel-1/LConn1
  brazo1fribracarbono-2/RConn2 -- Weld6/LConn1
  Weld6/RConn1 -- aumento-1/LConn1
  brazo1fribracarbono-1/RConn1 -- Weld4/LConn1
  Weld4/RConn1 -- aumento-2/LConn1
  aumento-1/RConn1 -- Weld19/LConn1
  Revolute2/RConn1 -- Copia de motordymaxixel^Ensamblaje1-2/RConn1
  aumento-2/RConn1 -- Weld20/LConn1
  Weld20/RConn1 -- Copia de motordymaxixel^Ensamblaje1-2/LConn1
